simulink model "Compressor"  (R2020a)
settings: Solver=VariableStepAuto  StartTime=0.0  StopTime=10.0  RelTol=1e-3
settings Model: Creator=YJT  LastModifiedBy=YJT

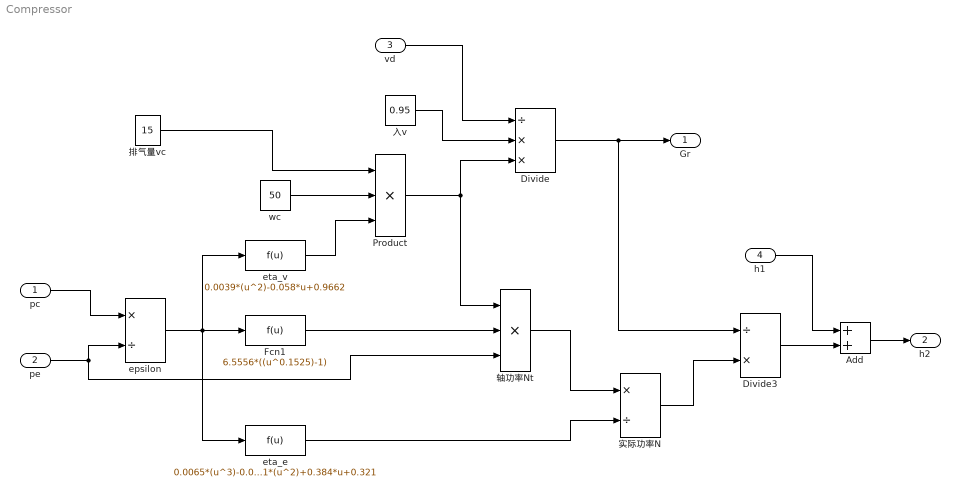
== system Compressor ==
  pc : Inport
  pe : Inport  Port=2
  vd : Inport  Port=3
  h1 : Inport  Port=4
  Add : Sum
  Divide : Product  Inputs=/**
  Divide3 : Product  Inputs=/*
  Fcn1 : Fcn  Expr=6.5556*((u^0.1525)-1)
  Product : Product  Inputs=3
  epsilon : Product  Inputs=*/
  eta_e : Fcn  Expr=0.0065*(u^3)-0.0901*(u^2)+0.384*u+0.321
  eta_v : Fcn  Expr=0.0039*(u^2)-0.058*u+0.9662
  wc : Constant  Value=50
  入v : Constant  Value=0.95
  实际功率N : Product  Inputs=*/
  排气量vc : Constant  Value=15
  轴功率Nt : Product  Inputs=3
  Gr : Outport
  h2 : Outport  Port=2
  wires:
  pc/1 -> epsilon/1
  pe/1 -> epsilon/2, 轴功率Nt/3
  epsilon/1 -> eta_e/1, eta_v/1, Fcn1/1
  eta_v/1 -> Product/3
  wc/1 -> Product/2
  排气量vc/1 -> Product/1
  vd/1 -> Divide/1
  入v/1 -> Divide/2
  Product/1 -> Divide/3, 轴功率Nt/1
  Fcn1/1 -> 轴功率Nt/2
  轴功率Nt/1 -> 实际功率N/1
  eta_e/1 -> 实际功率N/2
  实际功率N/1 -> Divide3/2
  Divide/1 -> Divide3/1, Gr/1
  Divide3/1 -> Add/2
  h1/1 -> Add/1
  Add/1 -> h2/1
